simulink model "SampleMissionProfile"  (Simulink 8.2)
settings: Solver=ode45  StartTime=0.0  StopTime=1000  RelTol=1e-3
undefined symbols (not defined in the file): del_P, del_rho, del_T, dens_msl, MSSN, pres_msl, temp_msl
settings Model: Creator=mwillms4  LastModifiedBy=ASELab1

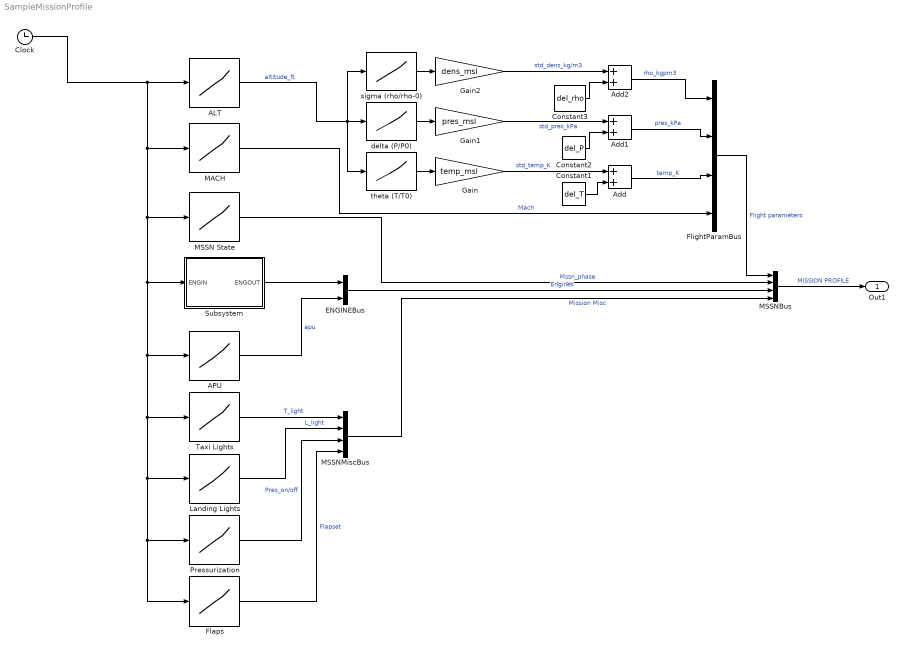
== system SampleMissionProfile ==
  ALT : Lookup  InputValues=MSSN.cond.time  Table=MSSN.cond.alt
  APU : Lookup  InputValues=MSSN.eng.time  Table=MSSN.eng.apu  LookUpMeth=Use Input Below
  Add : Sum
  Add1 : Sum
  Add2 : Sum
  Clock : Clock
  Constant1 : Constant  Value=del_T
  Constant2 : Constant  Value=del_P
  Constant3 : Constant  Value=del_rho
  ENGINEBus : BusCreator  Inputs=2
  Flaps : Lookup  InputValues=MSSN.el.time  Table=MSSN.el.flaps  LookUpMeth=Use Input Below
  FlightParamBus : BusCreator  OutDataTypeStr=Bus: MISSIONBUS
  Gain : Gain  Gain=temp_msl
  Gain1 : Gain  Gain=pres_msl
  Gain2 : Gain  Gain=dens_msl
  Landing Lights : Lookup  InputValues=MSSN.el.time  Table=MSSN.el.landinglit  LookUpMeth=Use Input Below
  MACH : Lookup  InputValues=MSSN.cond.time  Table=MSSN.cond.mach
  MSSN State : Lookup  InputValues=MSSN.gen.time  Table=MSSN.gen.state  LookUpMeth=Use Input Below
  MSSNBus : BusCreator
  MSSNMiscBus : BusCreator
  Pressurization : Lookup  InputValues=MSSN.pnu.time  Table=MSSN.pnu.pres  LookUpMeth=Use Input Below
  Subsystem : Subsystem
  Taxi Lights : Lookup  InputValues=MSSN.el.time  Table=MSSN.el.taxilit  LookUpMeth=Use Input Below
  delta (P/P0) : Lookup_n-D  NumberOfTableDimensions=1  BreakpointsForDimension1=|  Table=|  RndMeth=Simplest  InputSameDT=on
      BreakpointsForDimension1=|
      | [0
      | 1000
      | 2000
      | 3000
      | 4000
      | 5000
      | 6000
      | 7000
      | 8000
      | 9000
      | 10000
      | 11000
      | 12000
      | 13000
      | 14000
      | 15000
      | 16000
      | 17000
      | 18000
      | 19000
      | 20000
      | 21000
      | 22000
      | 23000
      | 24000
      | 25000
      | 26000
      | 27000
      | 28000
      | 29000
      | 30000
      | 31000
      | 32000
      | 33000
      | 34000
      | 35000
      | 36000
      | 37000
      | 38000
      | 39000
      | 40000
      | 41000
      | 42000
      | 43000
      | 44000
      | 45000
      | 46000
      | 47000
      | 48000
      | 49000
      | 50000
      | 51000
      | 52000
      | 53000
      | 54000
      | 55000
      | 56000
      | 57000
      | 58000
      | 59000
      | 60000
      | 61000
      | 62000
      | 63000
      | 64000
      | 65000
      | ]
      Table=|
      | [1
      | 0.9644
      | 0.9298
      | 0.8963
      | 0.8637
      | 0.8321
      | 0.8014
      | 0.7717
      | 0.7429
      | 0.7149
      | 0.6878
      | 0.6616
      | 0.6362
      | 0.6115
      | 0.5877
      | 0.5646
      | 0.5422
      | 0.5206
      | 0.4997
      | 0.4795
      | 0.4599
      | 0.441
      | 0.4227
      | 0.4051
      | 0.388
      | 0.3716
      | 0.3557
      | 0.3404
      | 0.3256
      | 0.3113
      | 0.2975
      | 0.2843
      | 0.2715
      | 0.2592
      | 0.2474
      | 0.236
      | 0.225
      | 0.2145
      | 0.2044
      | 0.1949
      | 0.1858
      | 0.1771
      | 0.1688
      | 0.1609
      | 0.1534
      | 0.1462
      | 0.1394
      | 0.1329
      | 0.1267
      | 0.1208
      | 0.1151
      | 0.1097
      | 0.1046
      | 0.0997
      | 0.0951
      | 0.0906
      | 0.0864
      | 0.0824
      | 0.0785
      | 0.0749
      | 0.0714
      | 0.068
      | 0.0649
      | 0.0618
      | 0.059
      | 0.0562
      | 
      | 
      | ]
  sigma (rho/rho-0) : Lookup_n-D  NumberOfTableDimensions=1  BreakpointsForDimension1=|  Table=|  RndMeth=Simplest  InputSameDT=on
      BreakpointsForDimension1=|
      | [0
      | 1000
      | 2000
      | 3000
      | 4000
      | 5000
      | 6000
      | 7000
      | 8000
      | 9000
      | 10000
      | 11000
      | 12000
      | 13000
      | 14000
      | 15000
      | 16000
      | 17000
      | 18000
      | 19000
      | 20000
      | 21000
      | 22000
      | 23000
      | 24000
      | 25000
      | 26000
      | 27000
      | 28000
      | 29000
      | 30000
      | 31000
      | 32000
      | 33000
      | 34000
      | 35000
      | 36000
      | 37000
      | 38000
      | 39000
      | 40000
      | 41000
      | 42000
      | 43000
      | 44000
      | 45000
      | 46000
      | 47000
      | 48000
      | 49000
      | 50000
      | 51000
      | 52000
      | 53000
      | 54000
      | 55000
      | 56000
      | 57000
      | 58000
      | 59000
      | 60000
      | 61000
      | 62000
      | 63000
      | 64000
      | 65000
      | ]
      Table=|
      | [1
      | 0.9711
      | 0.9428
      | 0.9151
      | 0.8881
      | 0.8617
      | 0.8359
      | 0.8107
      | 0.7861
      | 0.7621
      | 0.7386
      | 0.7157
      | 0.6933
      | 0.6715
      | 0.6502
      | 0.6295
      | 0.6092
      | 0.5895
      | 0.5702
      | 0.5514
      | 0.5332
      | 0.5153
      | 0.498
      | 0.4811
      | 0.4646
      | 0.4486
      | 0.433
      | 0.4178
      | 0.4031
      | 0.3887
      | 0.3747
      | 0.3611
      | 0.348
      | 0.3351
      | 0.3227
      | 0.3106
      | 0.2988
      | 0.2852
      | 0.2719
      | 0.2592
      | 0.2471
      | 0.2355
      | 0.2245
      | 0.214
      | 0.204
      | 0.1945
      | 0.1854
      | 0.1767
      | 0.1685
      | 0.1606
      | 0.1531
      | 0.146
      | 0.1391
      | 0.1326
      | 0.1264
      | 0.1205
      | 0.1149
      | 0.1096
      | 0.1044
      | 0.0996
      | 0.0949
      | 0.0905
      | 0.0863
      | 0.0822
      | 0.0784
      | 0.0747
      | 
      | ]
  theta (T/T0) : Lookup_n-D  NumberOfTableDimensions=1  BreakpointsForDimension1=|  Table=|  RndMeth=Simplest  InputSameDT=on
      BreakpointsForDimension1=|
      | [0
      | 1000
      | 2000
      | 3000
      | 4000
      | 5000
      | 6000
      | 7000
      | 8000
      | 9000
      | 10000
      | 11000
      | 12000
      | 13000
      | 14000
      | 15000
      | 16000
      | 17000
      | 18000
      | 19000
      | 20000
      | 21000
      | 22000
      | 23000
      | 24000
      | 25000
      | 26000
      | 27000
      | 28000
      | 29000
      | 30000
      | 31000
      | 32000
      | 33000
      | 34000
      | 35000
      | 36000
      | 37000
      | 38000
      | 39000
      | 40000
      | 41000
      | 42000
      | 43000
      | 44000
      | 45000
      | 46000
      | 47000
      | 48000
      | 49000
      | 50000
      | 51000
      | 52000
      | 53000
      | 54000
      | 55000
      | 56000
      | 57000
      | 58000
      | 59000
      | 60000
      | 61000
      | 62000
      | 63000
      | 64000
      | 65000
      | ]
      Table=|
      | [1
      | 0.9931
      | 0.9863
      | 0.9794
      | 0.9725
      | 0.9656
      | 0.9588
      | 0.9519
      | 0.945
      | 0.9381
      | 0.9313
      | 0.9244
      | 0.9175
      | 0.9107
      | 0.9038
      | 0.8969
      | 0.8901
      | 0.8832
      | 0.8763
      | 0.8695
      | 0.8626
      | 0.8558
      | 0.8489
      | 0.842
      | 0.8352
      | 0.8283
      | 0.8215
      | 0.8146
      | 0.8077
      | 0.8009
      | 0.794
      | 0.7872
      | 0.7803
      | 0.7735
      | 0.7666
      | 0.7598
      | 0.7529
      | 0.7519
      | 0.7519
      | 0.7519
      | 0.7519
      | 0.7519
      | 0.7519
      | 0.7519
      | 0.7519
      | 0.7519
      | 0.7519
      | 0.7519
      | 0.7519
      | 0.7519
      | 0.7519
      | 0.7519
      | 0.7519
      | 0.7519
      | 0.7519
      | 0.7519
      | 0.7519
      | 0.7519
      | 0.7519
      | 0.7519
      | 0.7519
      | 0.7519
      | 0.7519
      | 0.7519
      | 0.7519
      | 0.7519
      | 
      | ]
  Out1 : Outport
  wires:
  Clock/1 -> Pressurization/1, Flaps/1, Landing Lights/1, Taxi Lights/1, APU/1, Subsystem/1(ENGIN), MSSN State/1, MACH/1, ALT/1
  ENGINEBus/1 -> MSSNBus/3  "Engines"
  MSSNMiscBus/1 -> MSSNBus/4  "Mission Misc"
  Taxi Lights/1 -> MSSNMiscBus/1  "T_light"
  APU/1 -> ENGINEBus/2  "apu"
  Landing Lights/1 -> MSSNMiscBus/2  "L_light"
  Pressurization/1 -> MSSNMiscBus/3  "Pres_on/off"
  Flaps/1 -> MSSNMiscBus/4  "Flapset"
  MSSN State/1 -> MSSNBus/2  "Mssn_phase"
  ALT/1 -> delta (P/P0)/1, sigma (rho/rho-0)/1, theta (T/T0)/1  "altitude_ft"
  Constant1/1 -> Add/2
  Constant2/1 -> Add1/2
  Constant3/1 -> Add2/2
  Gain2/1 -> Add2/1  "std_dens_kg/m3"
  Gain1/1 -> Add1/1  "std_pres_kPa"
  Gain/1 -> Add/1  "std_temp_K"
  theta (T/T0)/1 -> Gain/1
  sigma (rho/rho-0)/1 -> Gain2/1
  delta (P/P0)/1 -> Gain1/1
  Add2/1 -> FlightParamBus/1  "rho_kgpm3"
  Add1/1 -> FlightParamBus/2  "pres_kPa"
  Add/1 -> FlightParamBus/3  "temp_K"
  MACH/1 -> FlightParamBus/4  "Mach"
  FlightParamBus/1 -> MSSNBus/1  "Flight parameters"
  Subsystem/1(ENGOUT) -> ENGINEBus/1
  MSSNBus/1 -> Out1/1  "MISSION PROFILE"

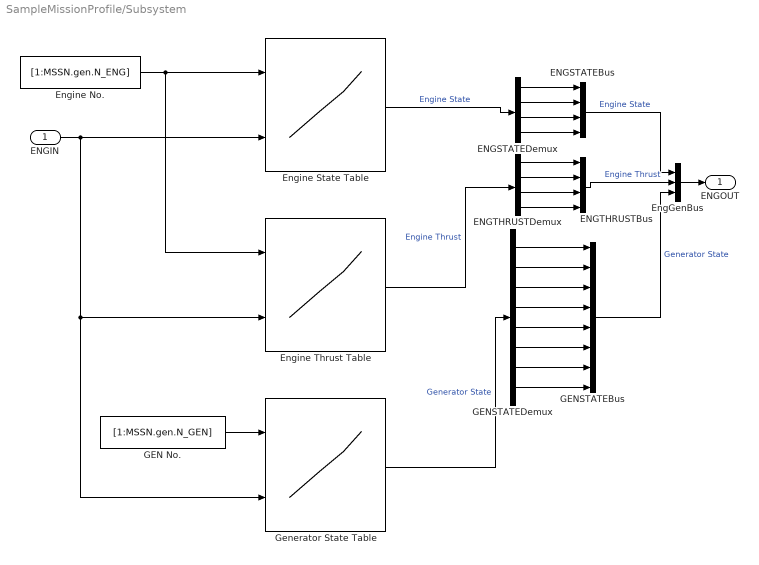
== system SampleMissionProfile/Subsystem ==
  ENGIN : Inport
  ENGSTATEBus : BusCreator
  ENGSTATEDemux : Demux
  ENGTHRUSTBus : BusCreator
  ENGTHRUSTDemux : Demux
  EngGenBus : BusCreator  Inputs=3
  Engine No. : Constant  Value=[1:MSSN.gen.N_ENG]
  Engine State Table : Lookup2D  RowIndex=[1:MSSN.gen.N_ENG]  ColumnIndex=MSSN.eng.time  Table=[MSSN.eng.Eng1;MSSN.eng.Eng2;MSSN.eng.Eng3;MSSN.eng.Eng4]  LookUpMeth=Use Input Below
  Engine Thrust Table : Lookup2D  RowIndex=[1:MSSN.gen.N_ENG]  ColumnIndex=MSSN.eng.time  Table=[MSSN.eng.EngThrust1;MSSN.eng.EngThrust2;MSSN.eng.EngThrust3;MSSN.eng.EngThrust4]  LookUpMeth=Use Input Below
  GEN No. : Constant  Value=[1:MSSN.gen.N_GEN]
  GENSTATEBus : BusCreator  Inputs=8
  GENSTATEDemux : Demux  Outputs=8
  Generator State Table : Lookup2D  RowIndex=[1:MSSN.gen.N_GEN]  ColumnIndex=MSSN.eng.time  Table=[MSSN.eng.Gen1;MSSN.eng.Gen2;MSSN.eng.Gen3;MSSN.eng.Gen4;MSSN.eng.Gen5;MSSN.eng.Gen6;MSSN.eng.Gen7;MSSN.eng.Gen8]  LookUpMeth=Use Input Below
  ENGOUT : Outport
  wires:
  ENGIN/1 -> Engine State Table/2, Engine Thrust Table/2, Generator State Table/2
  Engine No./1 -> Engine State Table/1, Engine Thrust Table/1
  Engine State Table/1 -> ENGSTATEDemux/1  "Engine State"
  Engine Thrust Table/1 -> ENGTHRUSTDemux/1  "Engine Thrust"
  ENGSTATEDemux/1 -> ENGSTATEBus/1
  ENGSTATEDemux/2 -> ENGSTATEBus/2
  ENGSTATEBus/1 -> EngGenBus/1  "Engine State"
  ENGTHRUSTDemux/1 -> ENGTHRUSTBus/1
  ENGTHRUSTDemux/2 -> ENGTHRUSTBus/2
  ENGTHRUSTBus/1 -> EngGenBus/2  "Engine Thrust"
  GENSTATEBus/1 -> EngGenBus/3  "Generator State"
  Generator State Table/1 -> GENSTATEDemux/1  "Generator State"
  EngGenBus/1 -> ENGOUT/1
  GEN No./1 -> Generator State Table/1
  GENSTATEDemux/1 -> GENSTATEBus/1
  GENSTATEDemux/2 -> GENSTATEBus/2
  GENSTATEDemux/3 -> GENSTATEBus/3
  GENSTATEDemux/4 -> GENSTATEBus/4
  GENSTATEDemux/5 -> GENSTATEBus/5
  GENSTATEDemux/6 -> GENSTATEBus/6
  GENSTATEDemux/7 -> GENSTATEBus/7
  GENSTATEDemux/8 -> GENSTATEBus/8
  ENGTHRUSTDemux/3 -> ENGTHRUSTBus/3
  ENGSTATEDemux/3 -> ENGSTATEBus/3
  ENGTHRUSTDemux/4 -> ENGTHRUSTBus/4
  ENGSTATEDemux/4 -> ENGSTATEBus/4
